simulink model "factorial_using_for"  (R2021b)
settings: Solver=VariableStepAuto  StartTime=1  StopTime=1  RelTol=1e-3
settings Model: Creator=Bhumil Depani  LastModifiedBy=Bhumil Depani

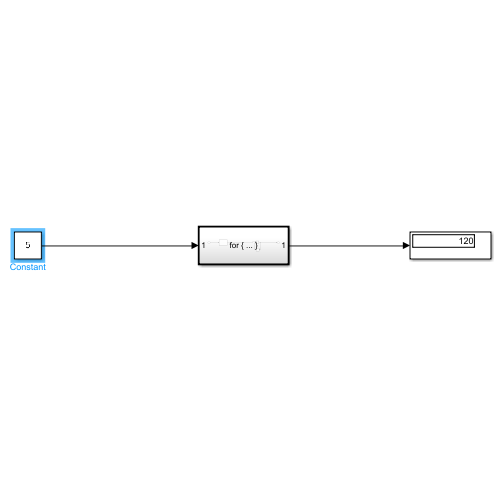
[thumbnail: Simulink's stored preview of the top-level diagram]
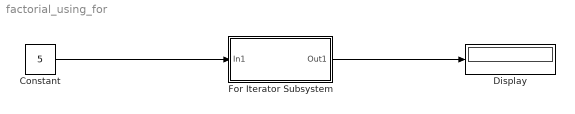
== system factorial_using_for ==
  Constant : Constant  Value=5
  Display : Display
  For Iterator Subsystem : Subsystem  TreatAsAtomicUnit=on
  wires:
  Constant/1 -> For Iterator Subsystem/1(In1)
  For Iterator Subsystem/1(Out1) -> Display/1

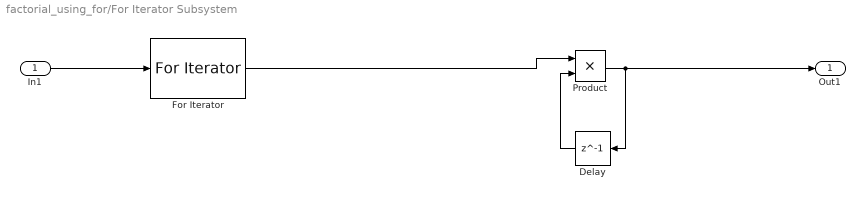
== system factorial_using_for/For Iterator Subsystem ==
  In1 : Inport
  Delay : Delay  DelayLength=1  InitialCondition=1
  For Iterator : ForIterator  IterationSource=external
  Product : Product  OutDataTypeStr=int32
  Out1 : Outport
  wires:
  In1/1 -> For Iterator/1
  For Iterator/1 -> Product/1
  Product/1 -> Delay/1, Out1/1
  Delay/1 -> Product/2
